simulink model "PFE_2Lignes_RNA (2)"  (R2024a)
settings: Solver=ode4  StartTime=0.0  StopTime=0.18  RelTol=1e-3
libraries: neural x202, spsRMSLib x12, spsThreePhasePISectionLineLib x4, spsThreePhaseFaultLib x2, spsThreePhaseVIMeasurementLib x2, spsThreePhaseSourceLib x2, spspowerguiLib x1
(part 3 of 10)

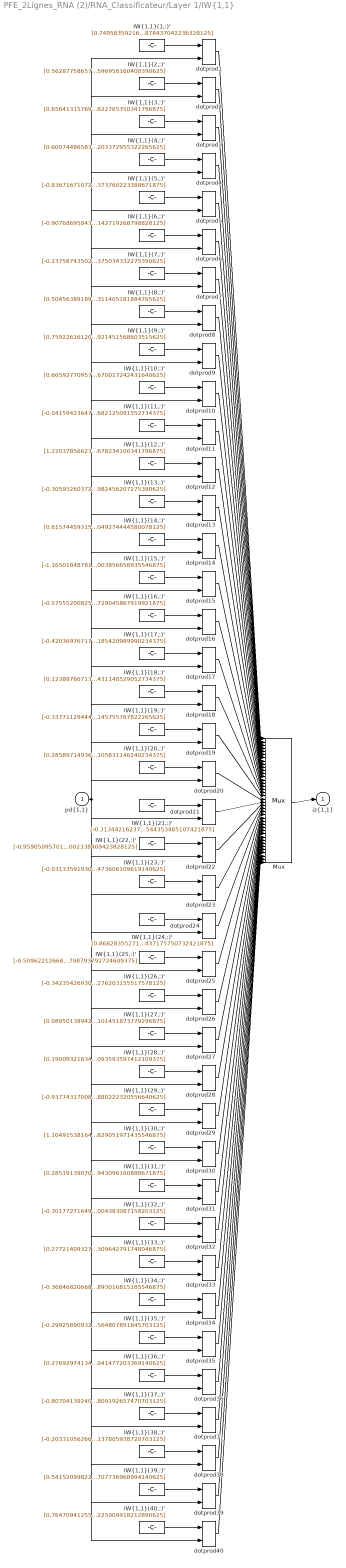
== system PFE_2Lignes_RNA (2)/RNA_Classificateur/Layer 1/IW{1,1} ==
  "pd{1,1}" : Inport  PortDimensions=12
      mask Display: e = 0.06;c1 = [120 230 180]/255;c2 = ([120 230 180]+0)/(256+128);c3 = ([120 230 180]+128)/(256+128);patch([0 1 1 0],[0 0 1 1],c1);patch([0 1 1 1-e 1-e 0+e],[0 0 1 1-e 0+e 0+e],c2);patch([0 0 1 1-e 0+e 0+e],[0 1 1 1-e 1-e 0+e],c3);plot([0 1 1 0 0],[0 0 1 1 0]);
  "IW{1,1}(1,:)'" : Constant  Value=[0.74958359216990821938253475309466011822223663330078125;-0.8029473672631188829740267465240322053432464599609375;-0.542336688026836544196385148097760975360870361328125;-0.787174648813282917814149186597205698490142822265625;0.5934798816135102850211069380748085677623748779296875;0.1866611157092597783613285855608410201966762542724609375;-0.408879266244710659616856673892471008002758026123046875;0.01913239052331479339574826781245064921677112579345703125;-0.106127660088452147046922391382395289838314056396484375;0.5668667292416820213674100159551016986370086669921875;-0.12326281029071710360067726242050412110984325408935546875;0.79123122581524285568121968026389367878437042236328125]
      mask Display: e = 0.06;c1 = [120 150 230]/255;c2 = ([120 150 230]+0)/383;c3 = ([120 150 230]+128)/383;patch([0 1 1 0],[0 0 1 1],c1);patch([0 1 1 1-e 1-e 0+e],[0 0 1 1-e 0+e 0+e],c2);patch([0 0 1 1-e 0+e 0+e],[0 1 1 1-e 1-e 0+e],c3);plot([0 1 1 0 0],[0 0 1 1 0]);disp('Weights');
  "IW{1,1}(10,:)'" : Constant  Value=[0.60592770957896824324251383586670272052288055419921875;-0.57064145847572245173751070979051291942596435546875;-0.57683424122696991265257793202181346714496612548828125;-1.4495291514928378973081635194830596446990966796875;-0.73466382714012545829262990082497708499431610107421875;-0.64755891681742239196495347641757689416408538818359375;-0.60153064759523289239950827322900295257568359375;-0.90205827349148481886231820681132376194000244140625;0.5948536687714207626953566432348452508449554443359375;-0.50297219156111128146591227050521411001682281494140625;1.567811975206783614567029871977865695953369140625;-0.252912599872824161995055192164727486670017242431640625]
      mask Display: e = 0.06;c1 = [120 150 230]/255;c2 = ([120 150 230]+0)/383;c3 = ([120 150 230]+128)/383;patch([0 1 1 0],[0 0 1 1],c1);patch([0 1 1 1-e 1-e 0+e],[0 0 1 1-e 0+e 0+e],c2);patch([0 0 1 1-e 0+e 0+e],[0 1 1 1-e 1-e 0+e],c3);plot([0 1 1 0 0],[0 0 1 1 0]);disp('Weights');
  "IW{1,1}(11,:)'" : Constant  Value=[-0.041594236471159569401567779323158902116119861602783203125;0.0541834052582221004090712312972755171358585357666015625;-1.2601601303957588040560722220106981694698333740234375;-2.32855835010428080522615346126258373260498046875;-1.3408389740320434402320870503899641335010528564453125;0.3734499673677518227776772619108669459819793701171875;0.5996288174482080624017044101492501795291900634765625;0.442299587174693920044177275485708378255367279052734375;-0.79910808052954729330252803265466354787349700927734375;-0.67576330904074810579373888685950078070163726806640625;1.6528925781939183270452531360206194221973419189453125;2.3480592220230303013295269920490682125091552734375]
      mask Display: e = 0.06;c1 = [120 150 230]/255;c2 = ([120 150 230]+0)/383;c3 = ([120 150 230]+128)/383;patch([0 1 1 0],[0 0 1 1],c1);patch([0 1 1 1-e 1-e 0+e],[0 0 1 1-e 0+e 0+e],c2);patch([0 0 1 1-e 0+e 0+e],[0 1 1 1-e 1-e 0+e],c3);plot([0 1 1 0 0],[0 0 1 1 0]);disp('Weights');
  "IW{1,1}(12,:)'" : Constant  Value=[1.2203785662394890376702960566035471856594085693359375;-0.08947721759545544661929028507074690423905849456787109375;-0.248432382462659473443267188486061058938503265380859375;-1.6836523036402055719662484989385120570659637451171875;1.8000899737378299736434428268694318830966949462890625;-0.324050010440849245441086168284527957439422607421875;1.327222054704254361467974376864731311798095703125;0.67379058195528285235553767051897011697292327880859375;-1.4433613727145309102439796333783306181430816650390625;-1.0976528220958334802759281956241466104984283447265625;0.2476851035413273616203611027231090702116489410400390625;1.6356974077387167465502670893329195678234100341796875]
      mask Display: e = 0.06;c1 = [120 150 230]/255;c2 = ([120 150 230]+0)/383;c3 = ([120 150 230]+128)/383;patch([0 1 1 0],[0 0 1 1],c1);patch([0 1 1 1-e 1-e 0+e],[0 0 1 1-e 0+e 0+e],c2);patch([0 0 1 1-e 0+e 0+e],[0 1 1 1-e 1-e 0+e],c3);plot([0 1 1 0 0],[0 0 1 1 0]);disp('Weights');
  "IW{1,1}(13,:)'" : Constant  Value=[-0.305952603724911120774976325265015475451946258544921875;0.2109724324184586163877241915542981587350368499755859375;-0.871724462567311508820466769975610077381134033203125;0.368499768652701009674643728430964983999729156494140625;0.246673658464245326715769124348298646509647369384765625;-0.442730444406182865879628707261872477829456329345703125;-1.096603408414358771238994449959136545658111572265625;0.434524950756032535270634298285585828125476837158203125;-0.3054258760453316678962210062309168279170989990234375;0.24218392291231183310884489401360042393207550048828125;0.8646470074893743973376558642485179007053375244140625;-0.1907281441165162017004064409775310195982456207275390625]
      mask Display: e = 0.06;c1 = [120 150 230]/255;c2 = ([120 150 230]+0)/383;c3 = ([120 150 230]+128)/383;patch([0 1 1 0],[0 0 1 1],c1);patch([0 1 1 1-e 1-e 0+e],[0 0 1 1-e 0+e 0+e],c2);patch([0 0 1 1-e 0+e 0+e],[0 1 1 1-e 1-e 0+e],c3);plot([0 1 1 0 0],[0 0 1 1 0]);disp('Weights');
  "IW{1,1}(14,:)'" : Constant  Value=[0.61574459315147722637817651047953404486179351806640625;-1.0623190979043048987051633957889862358570098876953125;0.394034092887489084677810069479164667427539825439453125;-2.248369712060643177409247073228470981121063232421875;0.5275119752705583753282780890003778040409088134765625;2.438367056160711143775188247673213481903076171875;0.22857017880371277573914312597480602562427520751953125;-1.0317290968902927961181603677687235176563262939453125;-0.2115671867019214003047267169677070342004299163818359375;-1.9027617943445609416386332668480463325977325439453125;0.60212334507071429978708465569070540368556976318359375;-0.82657639922626480188938558057998307049274444580078125]
      mask Display: e = 0.06;c1 = [120 150 230]/255;c2 = ([120 150 230]+0)/383;c3 = ([120 150 230]+128)/383;patch([0 1 1 0],[0 0 1 1],c1);patch([0 1 1 1-e 1-e 0+e],[0 0 1 1-e 0+e 0+e],c2);patch([0 0 1 1-e 0+e 0+e],[0 1 1 1-e 1-e 0+e],c3);plot([0 1 1 0 0],[0 0 1 1 0]);disp('Weights');
  "IW{1,1}(15,:)'" : Constant  Value=[-1.165018487811402270182270513032563030719757080078125;-0.1650855129048123537405245997433667071163654327392578125;-0.250310848664434038024495521312928758561611175537109375;0.367925209704279165823237462973338551819324493408203125;-1.053109213540988076118765093269757926464080810546875;1.1517107010752047902002459522918798029422760009765625;-0.5552091834027994554645601965603418648242950439453125;-0.56113154479276750041805144064710475504398345947265625;0.9146819847460303520847446634434163570404052734375;0.9900009386006491940435125798103399574756622314453125;-0.6463785661271843618891352889477275311946868896484375;-1.6172801313566320668968501195195131003856658935546875]
      mask Display: e = 0.06;c1 = [120 150 230]/255;c2 = ([120 150 230]+0)/383;c3 = ([120 150 230]+128)/383;patch([0 1 1 0],[0 0 1 1],c1);patch([0 1 1 1-e 1-e 0+e],[0 0 1 1-e 0+e 0+e],c2);patch([0 0 1 1-e 0+e 0+e],[0 1 1 1-e 1-e 0+e],c3);plot([0 1 1 0 0],[0 0 1 1 0]);disp('Weights');
  "IW{1,1}(16,:)'" : Constant  Value=[-0.57555200825379848605933830185676924884319305419921875;0.1994373147096829279600882500744774006307125091552734375;-0.412238082672211680890228535645292140543460845947265625;-0.42438555031721836297009531335788778960704803466796875;-0.93932452660136644961852425694814883172512054443359375;0.51360222841409786109778679019655101001262664794921875;0.1309899446070415252041385656411875970661640167236328125;-0.182257806815278977641270330423139967024326324462890625;0.8509013471342818935028162741218693554401397705078125;-0.388818754819776180031709600370959378778934478759765625;-1.025285492360808348166756331920623779296875;-0.203483170274558755608040883089415729045867919921875]
      mask Display: e = 0.06;c1 = [120 150 230]/255;c2 = ([120 150 230]+0)/383;c3 = ([120 150 230]+128)/383;patch([0 1 1 0],[0 0 1 1],c1);patch([0 1 1 1-e 1-e 0+e],[0 0 1 1-e 0+e 0+e],c2);patch([0 0 1 1-e 0+e 0+e],[0 1 1 1-e 1-e 0+e],c3);plot([0 1 1 0 0],[0 0 1 1 0]);disp('Weights');
  "IW{1,1}(17,:)'" : Constant  Value=[-0.420369767179770204013067314008367247879505157470703125;-0.64126174661276513777607988231466151773929595947265625;-0.388206694327405232858296812992193736135959625244140625;0.79635997694663307466811374979442916810512542724609375;0.60879685212660639148651853247429244220256805419921875;-0.591923664374563340828672153293155133724212646484375;0.1847453299443102270327443648056942038238048553466796875;-0.292667915200633343975056277486146427690982818603515625;-0.93611854779757319722222064228844828903675079345703125;0.2289312304159379085621850435927626676857471466064453125;0.477672003545131840240856035961769521236419677734375;-0.5429342609145473286247352007194422185420989990234375]
      mask Display: e = 0.06;c1 = [120 150 230]/255;c2 = ([120 150 230]+0)/383;c3 = ([120 150 230]+128)/383;patch([0 1 1 0],[0 0 1 1],c1);patch([0 1 1 1-e 1-e 0+e],[0 0 1 1-e 0+e 0+e],c2);patch([0 0 1 1-e 0+e 0+e],[0 1 1 1-e 1-e 0+e],c3);plot([0 1 1 0 0],[0 0 1 1 0]);disp('Weights');
  "IW{1,1}(18,:)'" : Constant  Value=[0.1238876071364114761497177141791325993835926055908203125;-0.77572554113254332808224944528774358332157135009765625;-0.08898063744331276281318565679612220264971256256103515625;1.57613590534866698789073780062608420848846435546875;0.2321005336110762706791632581371231935918331146240234375;-0.73676696655795925749998787068761885166168212890625;0.142658166835522681736847516731359064579010009765625;0.5747450524492887513616778960567899048328399658203125;-1.105370078416131551790613229968585073947906494140625;-2.21704492450396539737766943289898335933685302734375;1.0876593267347447469006738174357451498508453369140625;-0.72611976053770399541775759644224308431148529052734375]
      mask Display: e = 0.06;c1 = [120 150 230]/255;c2 = ([120 150 230]+0)/383;c3 = ([120 150 230]+128)/383;patch([0 1 1 0],[0 0 1 1],c1);patch([0 1 1 1-e 1-e 0+e],[0 0 1 1-e 0+e 0+e],c2);patch([0 0 1 1-e 0+e 0+e],[0 1 1 1-e 1-e 0+e],c3);plot([0 1 1 0 0],[0 0 1 1 0]);disp('Weights');
  "IW{1,1}(19,:)'" : Constant  Value=[-0.33771129444509118133765923630562610924243927001953125;0.0713367915505468130898947265450260601937770843505859375;0.2057896003228630033010659872161340899765491485595703125;2.20019744077431322892834941740147769451141357421875;-2.278663430987770244229295713012106716632843017578125;1.0768853464076302284269104347913525998592376708984375;-0.90948100032295198236198530139517970383167266845703125;1.2699892475521668000482122806715779006481170654296875;-0.374919053331535356843318140818155370652675628662109375;0.63267481864128505275601810353691689670085906982421875;-2.264524629934004718023743407684378325939178466796875;0.325611439903700505826833477840409614145755767822265625]
      mask Display: e = 0.06;c1 = [120 150 230]/255;c2 = ([120 150 230]+0)/383;c3 = ([120 150 230]+128)/383;patch([0 1 1 0],[0 0 1 1],c1);patch([0 1 1 1-e 1-e 0+e],[0 0 1 1-e 0+e 0+e],c2);patch([0 0 1 1-e 0+e 0+e],[0 1 1 1-e 1-e 0+e],c3);plot([0 1 1 0 0],[0 0 1 1 0]);disp('Weights');
  "IW{1,1}(2,:)'" : Constant  Value=[0.56287758657184328026090724961250089108943939208984375;0.62349868963765164853185751780983991920948028564453125;0.439815094086207059032034294432378374040126800537109375;0.47907287682830890229723763695801608264446258544921875;-0.209879774707502075870024782489053905010223388671875;-0.14745846190329292557663620755192823708057403564453125;-0.882701370669022100656775364768691360950469970703125;-0.7129252832091104163936279292101971805095672607421875;-0.76504800874029665891384865972213447093963623046875;-0.674348859168129255436952007585205137729644775390625;0.12273009441098824134908085170536651276051998138427734375;0.0229431755667083604743883284982075565494596958160400390625]
      mask Display: e = 0.06;c1 = [120 150 230]/255;c2 = ([120 150 230]+0)/383;c3 = ([120 150 230]+128)/383;patch([0 1 1 0],[0 0 1 1],c1);patch([0 1 1 1-e 1-e 0+e],[0 0 1 1-e 0+e 0+e],c2);patch([0 0 1 1-e 0+e 0+e],[0 1 1 1-e 1-e 0+e],c3);plot([0 1 1 0 0],[0 0 1 1 0]);disp('Weights');
  "IW{1,1}(20,:)'" : Constant  Value=[0.285897149366284797356030367154744453728199005126953125;-1.071211066211320339647272703587077558040618896484375;1.042160099435808451318052902934141457080841064453125;0.7370117529808191125795246989582665264606475830078125;-1.5106532728405495102919076089165173470973968505859375;-2.101314330452319634190416763885878026485443115234375;-0.0824484752168814782891104187001474201679229736328125;-1.1490974138089724565503502162755466997623443603515625;0.429340350947707449780210708922822959721088409423828125;1.6983804194670313325588040243019349873065948486328125;-0.6343565826158401588230617562658153474330902099609375;0.77783500854026621507131267208023928105831146240234375]
      mask Display: e = 0.06;c1 = [120 150 230]/255;c2 = ([120 150 230]+0)/383;c3 = ([120 150 230]+128)/383;patch([0 1 1 0],[0 0 1 1],c1);patch([0 1 1 1-e 1-e 0+e],[0 0 1 1-e 0+e 0+e],c2);patch([0 0 1 1-e 0+e 0+e],[0 1 1 1-e 1-e 0+e],c3);plot([0 1 1 0 0],[0 0 1 1 0]);disp('Weights');
  "IW{1,1}(21,:)'" : Constant  Value=[-0.313442162370461574472102483923663385212421417236328125;0.71069365723408439716735074398457072675228118896484375;0.7368025277872487510677501632017083466053009033203125;0.250940337360686938072973362068296410143375396728515625;0.36219419785523376820179919377551414072513580322265625;-0.045125177484137184158452527071858639828860759735107421875;-0.9373772040546857198251018417067825794219970703125;-0.8005469342332072191226188806467689573764801025390625;0.479706543742673463537329325845348648726940155029296875;-0.489203575067028051392981069511733949184417724609375;0.89499756815461750658613482301007024943828582763671875;-0.9393115987438498404316078449483029544353485107421875]
      mask Display: e = 0.06;c1 = [120 150 230]/255;c2 = ([120 150 230]+0)/383;c3 = ([120 150 230]+128)/383;patch([0 1 1 0],[0 0 1 1],c1);patch([0 1 1 1-e 1-e 0+e],[0 0 1 1-e 0+e 0+e],c2);patch([0 0 1 1-e 0+e 0+e],[0 1 1 1-e 1-e 0+e],c3);plot([0 1 1 0 0],[0 0 1 1 0]);disp('Weights');
  "IW{1,1}(22,:)'" : Constant  Value=[-0.9590509570193808119853429161594249308109283447265625;-0.493730940753906055729061108650057576596736907958984375;-0.8050191480991275572165477569797076284885406494140625;-0.28324115064341359726540758856572210788726806640625;-0.0855579308944639238543317105722962878644466400146484375;-0.2982589814017286844460841166437603533267974853515625;0.8651890058906144265193915998679585754871368408203125;-0.2127697372929893138149282094673253595829010009765625;-0.2118629696150977348434452096626046113669872283935546875;0.614617181476534657491583857336081564426422119140625;0.5175871796669948565750019042752683162689208984375;0.283420043030612689438640927619417198002338409423828125]
      mask Display: e = 0.06;c1 = [120 150 230]/255;c2 = ([120 150 230]+0)/383;c3 = ([120 150 230]+128)/383;patch([0 1 1 0],[0 0 1 1],c1);patch([0 1 1 1-e 1-e 0+e],[0 0 1 1-e 0+e 0+e],c2);patch([0 0 1 1-e 0+e 0+e],[0 1 1 1-e 1-e 0+e],c3);plot([0 1 1 0 0],[0 0 1 1 0]);disp('Weights');
  "IW{1,1}(23,:)'" : Constant  Value=[-0.031335919302591545843039710916855256073176860809326171875;-0.264118888374587523770742336637340486049652099609375;-0.99437742834595932439611942754709161818027496337890625;-0.48613182289601153396318977684131823480129241943359375;-0.65349579829228721106204602619982324540615081787109375;-0.82571376926229722581496162092662416398525238037109375;0.2174726698576462113887686200541793368756771087646484375;-0.73776313034045315486508798130671493709087371826171875;0.7378956287314346607075776773854158818721771240234375;-0.021332740476675084162483386762687587179243564605712890625;0.22149884534648800471501317588263191282749176025390625;0.86225703326549807403722525123157538473606109619140625]
      mask Display: e = 0.06;c1 = [120 150 230]/255;c2 = ([120 150 230]+0)/383;c3 = ([120 150 230]+128)/383;patch([0 1 1 0],[0 0 1 1],c1);patch([0 1 1 1-e 1-e 0+e],[0 0 1 1-e 0+e 0+e],c2);patch([0 0 1 1-e 0+e 0+e],[0 1 1 1-e 1-e 0+e],c3);plot([0 1 1 0 0],[0 0 1 1 0]);disp('Weights');
  "IW{1,1}(24,:)'" : Constant  Value=[0.8682835527171566258886059586075134575366973876953125;-0.338032804470147107966937483070068992674350738525390625;0.42663950553967155965295887654065154492855072021484375;0.07994886852322703740814091588617884553968906402587890625;-0.08234018636647570665854090066204662434756755828857421875;-0.56246234595990518556618553702719509601593017578125;-0.87800269121447815923175994612392969429492950439453125;0.67292433346952262862572524682036601006984710693359375;0.35843044089265407858846401722985319793224334716796875;-0.01037903761493451197661652685155786457471549510955810546875;0.419685343853191117347023464390076696872711181640625;0.82952182259364171112991925838286988437175750732421875]
      mask Display: e = 0.06;c1 = [120 150 230]/255;c2 = ([120 150 230]+0)/383;c3 = ([120 150 230]+128)/383;patch([0 1 1 0],[0 0 1 1],c1);patch([0 1 1 1-e 1-e 0+e],[0 0 1 1-e 0+e 0+e],c2);patch([0 0 1 1-e 0+e 0+e],[0 1 1 1-e 1-e 0+e],c3);plot([0 1 1 0 0],[0 0 1 1 0]);disp('Weights');
  "IW{1,1}(25,:)'" : Constant  Value=[-0.5096221266848035558183482862659730017185211181640625;-0.33408111078061530907490350728039629757404327392578125;0.053466115900446635478271417696305434219539165496826171875;-0.4334640772843945111247876411653123795986175537109375;-1.11725240942251868858647867455147206783294677734375;-0.8929572284339248877671479931450448930263519287109375;-0.2012255857319280305528508279166999273002147674560546875;-0.5698313421375633680554528837092220783233642578125;-0.7647545897762022537591519721900112926959991455078125;-0.25538460783435545931041588119114749133586883544921875;-0.353646046014701231907650935681886039674282073974609375;0.354005086921495182306074411826557479798793792724609375]
      mask Display: e = 0.06;c1 = [120 150 230]/255;c2 = ([120 150 230]+0)/383;c3 = ([120 150 230]+128)/383;patch([0 1 1 0],[0 0 1 1],c1);patch([0 1 1 1-e 1-e 0+e],[0 0 1 1-e 0+e 0+e],c2);patch([0 0 1 1-e 0+e 0+e],[0 1 1 1-e 1-e 0+e],c3);plot([0 1 1 0 0],[0 0 1 1 0]);disp('Weights');
  "IW{1,1}(26,:)'" : Constant  Value=[-0.3423542693008467807658234960399568080902099609375;-0.65877052593968421501102739057387225329875946044921875;0.393800774596241687230957495557959191501140594482421875;-1.1600315330827519755274579438264481723308563232421875;-0.71438883033852540460628688379074446856975555419921875;0.161594455696278116452191397911519743502140045166015625;-0.595002607394423232989311145502142608165740966796875;0.53582780307071098402360576073988340795040130615234375;-0.2830443249472971434244072952424176037311553955078125;0.2438679104402185771061084551547537557780742645263671875;0.8530165391517396944465190244955010712146759033203125;-0.477263046162692383678205487740342505276203155517578125]
      mask Display: e = 0.06;c1 = [120 150 230]/255;c2 = ([120 150 230]+0)/383;c3 = ([120 150 230]+128)/383;patch([0 1 1 0],[0 0 1 1],c1);patch([0 1 1 1-e 1-e 0+e],[0 0 1 1-e 0+e 0+e],c2);patch([0 0 1 1-e 0+e 0+e],[0 1 1 1-e 1-e 0+e],c3);plot([0 1 1 0 0],[0 0 1 1 0]);disp('Weights');
  "IW{1,1}(27,:)'" : Constant  Value=[0.08950138942217437942883151436035404913127422332763671875;1.3685401924282574182001326335011981427669525146484375;-0.288351551229408753496130657367757521569728851318359375;-0.71976588579313471871756746622850187122821807861328125;-0.52243867576969871269199074959033168852329254150390625;2.612100797819043140890471477177925407886505126953125;-1.27054609389886774550859627197496592998504638671875;1.4995893391046692944001961222966201603412628173828125;-0.099707396420515903567860505063435994088649749755859375;1.2431004909587823892280766813200898468494415283203125;-0.64312205526082066864290709418128244578838348388671875;-0.10866294126831392563570233278369414620101451873779296875]
      mask Display: e = 0.06;c1 = [120 150 230]/255;c2 = ([120 150 230]+0)/383;c3 = ([120 150 230]+128)/383;patch([0 1 1 0],[0 0 1 1],c1);patch([0 1 1 1-e 1-e 0+e],[0 0 1 1-e 0+e 0+e],c2);patch([0 0 1 1-e 0+e 0+e],[0 1 1 1-e 1-e 0+e],c3);plot([0 1 1 0 0],[0 0 1 1 0]);disp('Weights');
  "IW{1,1}(28,:)'" : Constant  Value=[0.190093216345575910519727358405361883342266082763671875;0.3459347222775852603859902956173755228519439697265625;0.1488544304146839636349142210747231729328632354736328125;-0.84436799503464687877141159333405084908008575439453125;-0.043616504441921312429375490182792418636381626129150390625;-0.406650868392631481551546812625019811093807220458984375;-0.6335629077808870857069223347934894263744354248046875;-0.1333311244937185613412822249301825650036334991455078125;-0.38599030556140478953608408119180239737033843994140625;-0.03760225945764107680080456930227228440344333648681640625;1.0547147290717828749251339104375801980495452880859375;-0.8816665448833267415551517842686735093593597412109375]
      mask Display: e = 0.06;c1 = [120 150 230]/255;c2 = ([120 150 230]+0)/383;c3 = ([120 150 230]+128)/383;patch([0 1 1 0],[0 0 1 1],c1);patch([0 1 1 1-e 1-e 0+e],[0 0 1 1-e 0+e 0+e],c2);patch([0 0 1 1-e 0+e 0+e],[0 1 1 1-e 1-e 0+e],c3);plot([0 1 1 0 0],[0 0 1 1 0]);disp('Weights');
  "IW{1,1}(29,:)'" : Constant  Value=[-0.9377431700885920928811856356333009898662567138671875;-0.41871014072329704180930320944753475487232208251953125;-0.30656734193459700410500090583809651434421539306640625;0.48579727512091064323129785407218150794506072998046875;0.568634796685665744320203884853981435298919677734375;0.041760693543964326479578375028722803108394145965576171875;0.50950195077496907014591442930395714938640594482421875;0.62995217911531053989193651432287879288196563720703125;0.465545832022614458622911115526221692562103271484375;0.93160272044449976558411208316101692616939544677734375;0.455869667774234266222066480622743256390094757080078125;0.07025705649596970803205664424240239895880222320556640625]
      mask Display: e = 0.06;c1 = [120 150 230]/255;c2 = ([120 150 230]+0)/383;c3 = ([120 150 230]+128)/383;patch([0 1 1 0],[0 0 1 1],c1);patch([0 1 1 1-e 1-e 0+e],[0 0 1 1-e 0+e 0+e],c2);patch([0 0 1 1-e 0+e 0+e],[0 1 1 1-e 1-e 0+e],c3);plot([0 1 1 0 0],[0 0 1 1 0]);disp('Weights');
  "IW{1,1}(3,:)'" : Constant  Value=[0.65641315769168706584224537436966784298419952392578125;0.95965783508391699907491556587046943604946136474609375;-0.2152247721630420607130673715801094658672809600830078125;0.317281125122891249912271405264618806540966033935546875;-0.61078832199027666138846370813553221523761749267578125;0.10949722031622351192670095088033122010529041290283203125;0.1124212875620385909680720715186907909810543060302734375;0.74937070531208183066240735570318065583705902099609375;0.7614081896496200929647102384478785097599029541015625;-0.416611934081368151527868803896126337349414825439453125;0.7932555092323492207384560970240272581577301025390625;0.89911069595746351268417129176668822765350341796875]
      mask Display: e = 0.06;c1 = [120 150 230]/255;c2 = ([120 150 230]+0)/383;c3 = ([120 150 230]+128)/383;patch([0 1 1 0],[0 0 1 1],c1);patch([0 1 1 1-e 1-e 0+e],[0 0 1 1-e 0+e 0+e],c2);patch([0 0 1 1-e 0+e 0+e],[0 1 1 1-e 1-e 0+e],c3);plot([0 1 1 0 0],[0 0 1 1 0]);disp('Weights');
  "IW{1,1}(30,:)'" : Constant  Value=[1.1049153816467895961039857866126112639904022216796875;-0.53997558976443393863320352465962059795856475830078125;-0.29341557443190480203298875494510866701602935791015625;-1.281561303027391129916168210911564528942108154296875;-1.5163694776935543462315081342239864170551300048828125;2.712509809409909156130424889852292835712432861328125;0.492131681291292644164769853887264616787433624267578125;0.174527918481056143473750807970645837485790252685546875;-0.349498727995869173934551099591772072017192840576171875;0.59797003361281808597738063326687552034854888916015625;0.83240948658350488731372252004803158342838287353515625;-0.05640705661161364570244103333607199601829051971435546875]
      mask Display: e = 0.06;c1 = [120 150 230]/255;c2 = ([120 150 230]+0)/383;c3 = ([120 150 230]+128)/383;patch([0 1 1 0],[0 0 1 1],c1);patch([0 1 1 1-e 1-e 0+e],[0 0 1 1-e 0+e 0+e],c2);patch([0 0 1 1-e 0+e 0+e],[0 1 1 1-e 1-e 0+e],c3);plot([0 1 1 0 0],[0 0 1 1 0]);disp('Weights');
  "IW{1,1}(31,:)'" : Constant  Value=[0.28519139070568699789731681448756717145442962646484375;-1.862443606980191734834306771517731249332427978515625;0.8013557171435683468274646656936965882778167724609375;1.1042674905459006762242779586813412606716156005859375;0.16541559268416694550296597299166023731231689453125;0.1831329137039820753596330860091256909072399139404296875;0.451396702089381818279179015007684938609600067138671875;-0.222687383867321175845432890127995051443576812744140625;1.629423175853772054466617191792465746402740478515625;-0.57012463147081238190594376646913588047027587890625;2.21204921457433467679720706655643880367279052734375;-2.8511850436189671853526306222192943096160888671875]
      mask Display: e = 0.06;c1 = [120 150 230]/255;c2 = ([120 150 230]+0)/383;c3 = ([120 150 230]+128)/383;patch([0 1 1 0],[0 0 1 1],c1);patch([0 1 1 1-e 1-e 0+e],[0 0 1 1-e 0+e 0+e],c2);patch([0 0 1 1-e 0+e 0+e],[0 1 1 1-e 1-e 0+e],c3);plot([0 1 1 0 0],[0 0 1 1 0]);disp('Weights');
  "IW{1,1}(32,:)'" : Constant  Value=[-0.301772716498337700841148034669458866119384765625;-0.414429934390460219528762308982550166547298431396484375;0.1380777058785409849850367436374654062092304229736328125;-0.7143244134519781685099815149442292749881744384765625;-0.77940794840309080004914221717626787722110748291015625;-1.2428186126836837654963119348394684493541717529296875;-0.391212337652795338893696452942094765603542327880859375;0.475034841084361392216095509866136126220226287841796875;-0.4299337892150332240959187402040697634220123291015625;-0.6281549902762579851156488075503148138523101806640625;1.060508076003738864301340072415769100189208984375;0.485821416719840915021677574259229004383087158203125]
      mask Display: e = 0.06;c1 = [120 150 230]/255;c2 = ([120 150 230]+0)/383;c3 = ([120 150 230]+128)/383;patch([0 1 1 0],[0 0 1 1],c1);patch([0 1 1 1-e 1-e 0+e],[0 0 1 1-e 0+e 0+e],c2);patch([0 0 1 1-e 0+e 0+e],[0 1 1 1-e 1-e 0+e],c3);plot([0 1 1 0 0],[0 0 1 1 0]);disp('Weights');
  "IW{1,1}(33,:)'" : Constant  Value=[0.277214093272214301411082715276279486715793609619140625;-0.92575351685280027336233388268738053739070892333984375;-0.94168797078716626192118610561010427772998809814453125;0.434861051287833533240956285226275213062763214111328125;-0.580249336840946927651430087280459702014923095703125;-0.379448799341846887411833222358836792409420013427734375;-0.008056916678392180009016243502628640271723270416259765625;0.838796765298734481319797851028852164745330810546875;-0.1206418706210981850457386599373421631753444671630859375;-0.1670855221535699486334891616934328339993953704833984375;-0.476500419080890302847564043986494652926921844482421875;0.529235878067051412898536000284366309642791748046875]
      mask Display: e = 0.06;c1 = [120 150 230]/255;c2 = ([120 150 230]+0)/383;c3 = ([120 150 230]+128)/383;patch([0 1 1 0],[0 0 1 1],c1);patch([0 1 1 1-e 1-e 0+e],[0 0 1 1-e 0+e 0+e],c2);patch([0 0 1 1-e 0+e 0+e],[0 1 1 1-e 1-e 0+e],c3);plot([0 1 1 0 0],[0 0 1 1 0]);disp('Weights');
  "IW{1,1}(34,:)'" : Constant  Value=[-0.3684682066801336919326104180072434246540069580078125;-0.6352643746280903780387916413019411265850067138671875;0.70922280885724386934043650398962199687957763671875;0.57918446406515367019807172255241312086582183837890625;-0.0775289597604681690601324817180284298956394195556640625;0.7739422565547275922881453880108892917633056640625;0.69494552120529384797720240385388024151325225830078125;-0.319218125764637761232478396777878515422344207763671875;0.57296390287849618960791531208087690174579620361328125;-0.0858820073557324814572666582535021007061004638671875;-0.056006971209040086467911834233746048994362354278564453125;0.859022811903467964356195807340554893016815185546875]
      mask Display: e = 0.06;c1 = [120 150 230]/255;c2 = ([120 150 230]+0)/383;c3 = ([120 150 230]+128)/383;patch([0 1 1 0],[0 0 1 1],c1);patch([0 1 1 1-e 1-e 0+e],[0 0 1 1-e 0+e 0+e],c2);patch([0 0 1 1-e 0+e 0+e],[0 1 1 1-e 1-e 0+e],c3);plot([0 1 1 0 0],[0 0 1 1 0]);disp('Weights');
  "IW{1,1}(35,:)'" : Constant  Value=[-0.299258909321519162016755899458075873553752899169921875;0.2966388415741152417837156463065184652805328369140625;1.018171120787297656562486736220307648181915283203125;-1.124625556509126766968620358966290950775146484375;-1.439779048212390666350302126375027000904083251953125;0.86076943642049152938255929257138632237911224365234375;-0.83449722454053343323465696812490932643413543701171875;0.85754039690351591129768848986714147031307220458984375;-0.50045011901598346337749489975976757705211639404296875;0.243723327944616041662584393634460866451263427734375;1.16440210158013979224733702722005546092987060546875;-0.586932156418353390137099268031306564807891845703125]
      mask Display: e = 0.06;c1 = [120 150 230]/255;c2 = ([120 150 230]+0)/383;c3 = ([120 150 230]+128)/383;patch([0 1 1 0],[0 0 1 1],c1);patch([0 1 1 1-e 1-e 0+e],[0 0 1 1-e 0+e 0+e],c2);patch([0 0 1 1-e 0+e 0+e],[0 1 1 1-e 1-e 0+e],c3);plot([0 1 1 0 0],[0 0 1 1 0]);disp('Weights');
  "IW{1,1}(36,:)'" : Constant  Value=[0.27692974134838854727291845847503282129764556884765625;0.77329622179783275015552135300822556018829345703125;-0.1675059555554003765109882806427776813507080078125;-0.89453860910611260326419369448558427393436431884765625;0.135909151123754623480266445767483673989772796630859375;-0.395709438384614475836542624165304005146026611328125;0.429729256934494541209090812117210589349269866943359375;0.74666018683282786572164013705332763493061065673828125;-0.3527021687177949171854152154992334544658660888671875;0.3362811681978075117882553968229331076145172119140625;-0.89909554477031738972669927534298039972782135009765625;-0.21445098130394557589539772379794158041477203369140625]
      mask Display: e = 0.06;c1 = [120 150 230]/255;c2 = ([120 150 230]+0)/383;c3 = ([120 150 230]+128)/383;patch([0 1 1 0],[0 0 1 1],c1);patch([0 1 1 1-e 1-e 0+e],[0 0 1 1-e 0+e 0+e],c2);patch([0 0 1 1-e 0+e 0+e],[0 1 1 1-e 1-e 0+e],c3);plot([0 1 1 0 0],[0 0 1 1 0]);disp('Weights');
  "IW{1,1}(37,:)'" : Constant  Value=[-0.80704139240025274393275367401656694710254669189453125;-0.25956215745037225506308686817646957933902740478515625;0.062075476078189729955969511365765356458723545074462890625;-0.325749693859563371756138394630397669970989227294921875;0.048574291467453123427588934646337293088436126708984375;0.89002497988019191321740208877599798142910003662109375;0.65323639460772664477872240240685641765594482421875;0.473597836610536393475712202416616491973400115966796875;-0.6069538552713442669528376427479088306427001953125;0.71567198082631888755855698036612011492252349853515625;-0.57652578697549572428471265084226615726947784423828125;0.0968309675838574801520763912776601500809192657470703125]
      mask Display: e = 0.06;c1 = [120 150 230]/255;c2 = ([120 150 230]+0)/383;c3 = ([120 150 230]+128)/383;patch([0 1 1 0],[0 0 1 1],c1);patch([0 1 1 1-e 1-e 0+e],[0 0 1 1-e 0+e 0+e],c2);patch([0 0 1 1-e 0+e 0+e],[0 1 1 1-e 1-e 0+e],c3);plot([0 1 1 0 0],[0 0 1 1 0]);disp('Weights');
  "IW{1,1}(38,:)'" : Constant  Value=[-0.203310562661204674572701378565398044884204864501953125;0.1788840987199529497519989718057331629097461700439453125;0.59513101026308756757998708053492009639739990234375;0.62350590814322259802793269045650959014892578125;1.8690381951598677989778707342338748276233673095703125;0.033032499657993895370022841007084934972226619720458984375;0.1757252254517237821662689611912355758249759674072265625;0.376049872023515752150757407434866763651371002197265625;0.69247672917727165486923013304476626217365264892578125;-1.2965395534711678937611623041448183357715606689453125;-0.93997399702286477118917673578835092484951019287109375;-0.6158625098382881635217245275271125137805938720703125]
      mask Display: e = 0.06;c1 = [120 150 230]/255;c2 = ([120 150 230]+0)/383;c3 = ([120 150 230]+128)/383;patch([0 1 1 0],[0 0 1 1],c1);patch([0 1 1 1-e 1-e 0+e],[0 0 1 1-e 0+e 0+e],c2);patch([0 0 1 1-e 0+e 0+e],[0 1 1 1-e 1-e 0+e],c3);plot([0 1 1 0 0],[0 0 1 1 0]);disp('Weights');
  "IW{1,1}(39,:)'" : Constant  Value=[0.54152099822578259047389792613103054463863372802734375;0.160174799891083907699140809199889190495014190673828125;-0.265786400862816851731196265973267145454883575439453125;-0.438811475002850170934465268146595917642116546630859375;0.39802426181648675740376575049594976007938385009765625;-0.686630434166221714775701912003569304943084716796875;-0.6962055175771599824230406738934107124805450439453125;1.040406774592970595705310188350267708301544189453125;-0.1016401613938503756262576871449709869921207427978515625;-0.10287828002409356298318954259229940362274646759033203125;-0.89655346696509052861756572383455932140350341796875;0.1339360030076012508803984246696927584707736968994140625]
      mask Display: e = 0.06;c1 = [120 150 230]/255;c2 = ([120 150 230]+0)/383;c3 = ([120 150 230]+128)/383;patch([0 1 1 0],[0 0 1 1],c1);patch([0 1 1 1-e 1-e 0+e],[0 0 1 1-e 0+e 0+e],c2);patch([0 0 1 1-e 0+e 0+e],[0 1 1 1-e 1-e 0+e],c3);plot([0 1 1 0 0],[0 0 1 1 0]);disp('Weights');
  "IW{1,1}(4,:)'" : Constant  Value=[0.600744865837338437586367945186793804168701171875;0.81736400318501434281159845340880565345287322998046875;0.96733501205360805652588851444306783378124237060546875;-0.60862859040623795703339737883652560412883758544921875;-0.89272101877643417200403064271085895597934722900390625;0.1445345695507280481262313287516008131206035614013671875;0.740054999198556995310127604170702397823333740234375;0.040437384319956602707346604574922821484506130218505859375;-0.1211526191911180549976023712588357739150524139404296875;-0.15047732920444889526123688483494333922863006591796875;-0.374151436983826968241118038349668495357036590576171875;-0.83178145689704996446067752913222648203372955322265625]
      mask Display: e = 0.06;c1 = [120 150 230]/255;c2 = ([120 150 230]+0)/383;c3 = ([120 150 230]+128)/383;patch([0 1 1 0],[0 0 1 1],c1);patch([0 1 1 1-e 1-e 0+e],[0 0 1 1-e 0+e 0+e],c2);patch([0 0 1 1-e 0+e 0+e],[0 1 1 1-e 1-e 0+e],c3);plot([0 1 1 0 0],[0 0 1 1 0]);disp('Weights');
  "IW{1,1}(40,:)'" : Constant  Value=[0.76470941255774160794089766568504273891448974609375;0.7509352048436939153219782383530400693416595458984375;0.66737230266155267432992559406557120382785797119140625;0.48756201808471200109806886757723987102508544921875;-0.58779814708604904982536254465230740606784820556640625;-0.290634263261388692267672695379587821662425994873046875;-0.52771118724632148921926955154049210250377655029296875;-0.3148389528275117310585073937545530498027801513671875;0.57937948246702497545612686735694296658039093017578125;-0.171738803664202688281648079282604157924652099609375;0.3012940300772226631664807428023777902126312255859375;0.55218816944886450759355511763715185225009918212890625]
      mask Display: e = 0.06;c1 = [120 150 230]/255;c2 = ([120 150 230]+0)/383;c3 = ([120 150 230]+128)/383;patch([0 1 1 0],[0 0 1 1],c1);patch([0 1 1 1-e 1-e 0+e],[0 0 1 1-e 0+e 0+e],c2);patch([0 0 1 1-e 0+e 0+e],[0 1 1 1-e 1-e 0+e],c3);plot([0 1 1 0 0],[0 0 1 1 0]);disp('Weights');
  "IW{1,1}(5,:)'" : Constant  Value=[-0.836716710720950995749944922863505780696868896484375;0.439411125451092399174513047910295426845550537109375;-0.1971139720063680711437115178341628052294254302978515625;-1.1003131078183823188254564229282550513744354248046875;0.02851888725345029518276618318850523792207241058349609375;-2.07109382987704382372839972958900034427642822265625;0.041456430285719471362515520240776822902262210845947265625;-0.65475871116475203859152998120407573878765106201171875;0.73798542834985292326877015511854551732540130615234375;1.375145340437987417914200705126859247684478759765625;1.914784300795295823860442396835424005985260009765625;0.95842545149267521775726663690875284373760223388671875]
      mask Display: e = 0.06;c1 = [120 150 230]/255;c2 = ([120 150 230]+0)/383;c3 = ([120 150 230]+128)/383;patch([0 1 1 0],[0 0 1 1],c1);patch([0 1 1 1-e 1-e 0+e],[0 0 1 1-e 0+e 0+e],c2);patch([0 0 1 1-e 0+e 0+e],[0 1 1 1-e 1-e 0+e],c3);plot([0 1 1 0 0],[0 0 1 1 0]);disp('Weights');
  "IW{1,1}(6,:)'" : Constant  Value=[-0.90768695843270974510375026511610485613346099853515625;-0.68351866834691554775105259977863170206546783447265625;1.2551835000960258614810527433292008936405181884765625;0.70545498306578269254174529123702086508274078369140625;-2.12807959265498336520749944611452519893646240234375;0.497168630609090722582976695775869302451610565185546875;-0.208328719791111061088173528332845307886600494384765625;0.1446092901230397742562416851797024719417095184326171875;-0.20704854405500150438257378482376225292682647705078125;2.448444622861401409608106405357830226421356201171875;-0.84050738810234004727561796244117431342601776123046875;0.039472385311477516112166341599731822498142719268798828125]
      mask Display: e = 0.06;c1 = [120 150 230]/255;c2 = ([120 150 230]+0)/383;c3 = ([120 150 230]+128)/383;patch([0 1 1 0],[0 0 1 1],c1);patch([0 1 1 1-e 1-e 0+e],[0 0 1 1-e 0+e 0+e],c2);patch([0 0 1 1-e 0+e 0+e],[0 1 1 1-e 1-e 0+e],c3);plot([0 1 1 0 0],[0 0 1 1 0]);disp('Weights');
  "IW{1,1}(7,:)'" : Constant  Value=[-0.237587435025801596566452644765377044677734375;0.94238608006865531852014328251243568956851959228515625;0.7885322751371912630702354363165795803070068359375;-0.1640548008439850768969137106978450901806354522705078125;-0.89611334097657946440307341617881320416927337646484375;0.0029081416154285743592977642180130715132690966129302978515625;-0.49500699678215998034147560247220098972320556640625;-0.457738654151404744663267365467618219554424285888671875;-0.354984270142353341981333869625814259052276611328125;-0.477987001565870428532178948444197885692119598388671875;0.00767064224277644833571709881425704224966466426849365234375;0.5465390990314862307286603027023375034332275390625]
      mask Display: e = 0.06;c1 = [120 150 230]/255;c2 = ([120 150 230]+0)/383;c3 = ([120 150 230]+128)/383;patch([0 1 1 0],[0 0 1 1],c1);patch([0 1 1 1-e 1-e 0+e],[0 0 1 1-e 0+e 0+e],c2);patch([0 0 1 1-e 0+e 0+e],[0 1 1 1-e 1-e 0+e],c3);plot([0 1 1 0 0],[0 0 1 1 0]);disp('Weights');
  "IW{1,1}(8,:)'" : Constant  Value=[0.50456389189707928633055189493461512029170989990234375;-0.765140951858942042207445410895161330699920654296875;0.1570690731750348512196779893201892264187335968017578125;0.2681208325762696187410938364337198436260223388671875;-0.82779326613658554823160784508218057453632354736328125;0.356993742779236511442064738730550743639469146728515625;-0.976280129291541509672924803453497588634490966796875;0.16504117848556243419722022736095823347568511962890625;0.356943967948731566419695582226268015801906585693359375;0.66842971143415164103629422243102453649044036865234375;0.449339961286215394675735979035380296409130096435546875;0.14220062142668743465634406675235368311405181884765625]
      mask Display: e = 0.06;c1 = [120 150 230]/255;c2 = ([120 150 230]+0)/383;c3 = ([120 150 230]+128)/383;patch([0 1 1 0],[0 0 1 1],c1);patch([0 1 1 1-e 1-e 0+e],[0 0 1 1-e 0+e 0+e],c2);patch([0 0 1 1-e 0+e 0+e],[0 1 1 1-e 1-e 0+e],c3);plot([0 1 1 0 0],[0 0 1 1 0]);disp('Weights');
  "IW{1,1}(9,:)'" : Constant  Value=[0.7592261612055779540497724156011827290058135986328125;0.046598748903399343779252461672513163648545742034912109375;-0.600588424610740911901984873111359775066375732421875;-0.94958054894314758431761447354801930487155914306640625;-1.3227754501645507811957713784067891538143157958984375;-0.77956703475742183950814023774000816047191619873046875;-0.50440860122289254974248251528479158878326416015625;-0.143701090065957270969221326595288701355457305908203125;0.726324471940543059389483460108749568462371826171875;0.648351302048403521638419988448731601238250732421875;0.6303467404820641828422367325401864945888519287109375;1.24140275687570156293304535211063921451568603515625]
      mask Display: e = 0.06;c1 = [120 150 230]/255;c2 = ([120 150 230]+0)/383;c3 = ([120 150 230]+128)/383;patch([0 1 1 0],[0 0 1 1],c1);patch([0 1 1 1-e 1-e 0+e],[0 0 1 1-e 0+e 0+e],c2);patch([0 0 1 1-e 0+e 0+e],[0 1 1 1-e 1-e 0+e],c3);plot([0 1 1 0 0],[0 0 1 1 0]);disp('Weights');
  Mux : Mux  Inputs=40
      mask Display: e = 0.06;c1 = [120 150 230]/255;c2 = ([120 150 230]+0)/383;c3 = ([120 150 230]+128)/383;patch([0 1 1 0],[0 0 1 1],c1);patch([0 1 1 1-e 1-e 0+e],[0 0 1 1-e 0+e 0+e],c2);patch([0 0 1 1-e 0+e 0+e],[0 1 1 1-e 1-e 0+e],c3);plot([0 1 1 0 0],[0 0 1 1 0]);disp('Mux');
  dotprod{1..40} (40 alike) : neural/Weight Functions/dotprod
  "iz{1,1}" : Outport
      mask Display: e = 0.06;c1 = [120 230 180]/255;c2 = ([120 230 180]+0)/(256+128);c3 = ([120 230 180]+128)/(256+128);patch([0 1 1 0],[0 0 1 1],c1);patch([0 1 1 1-e 1-e 0+e],[0 0 1 1-e 0+e 0+e],c2);patch([0 0 1 1-e 0+e 0+e],[0 1 1 1-e 1-e 0+e],c3);plot([0 1 1 0 0],[0 0 1 1 0]);
  wires:
  "IW{1,1}(1,:)'"/1 -> dotprod1/1
  "pd{1,1}"/1 -> dotprod1/2, dotprod2/2, dotprod3/2, dotprod4/2, dotprod5/2, dotprod6/2, dotprod7/2, dotprod8/2, dotprod9/2, dotprod10/2, dotprod11/2, dotprod12/2, dotprod13/2, dotprod14/2, dotprod15/2, dotprod16/2, dotprod17/2, dotprod18/2, dotprod19/2, dotprod20/2, dotprod21/2, dotprod22/2, dotprod23/2, dotprod24/2, dotprod25/2, dotprod26/2, dotprod27/2, dotprod28/2, dotprod29/2, dotprod30/2, dotprod31/2, dotprod32/2, dotprod33/2, dotprod34/2, dotprod35/2, dotprod36/2, dotprod37/2, dotprod38/2, dotprod39/2, dotprod40/2
  dotprod1/1 -> Mux/1
  "IW{1,1}(2,:)'"/1 -> dotprod2/1
  dotprod2/1 -> Mux/2
  "IW{1,1}(3,:)'"/1 -> dotprod3/1
  dotprod3/1 -> Mux/3
  "IW{1,1}(4,:)'"/1 -> dotprod4/1
  dotprod4/1 -> Mux/4
  "IW{1,1}(5,:)'"/1 -> dotprod5/1
  dotprod5/1 -> Mux/5
  "IW{1,1}(6,:)'"/1 -> dotprod6/1
  dotprod6/1 -> Mux/6
  "IW{1,1}(7,:)'"/1 -> dotprod7/1
  dotprod7/1 -> Mux/7
  "IW{1,1}(8,:)'"/1 -> dotprod8/1
  dotprod8/1 -> Mux/8
  "IW{1,1}(9,:)'"/1 -> dotprod9/1
  dotprod9/1 -> Mux/9
  "IW{1,1}(10,:)'"/1 -> dotprod10/1
  dotprod10/1 -> Mux/10
  "IW{1,1}(11,:)'"/1 -> dotprod11/1
  dotprod11/1 -> Mux/11
  "IW{1,1}(12,:)'"/1 -> dotprod12/1
  dotprod12/1 -> Mux/12
  "IW{1,1}(13,:)'"/1 -> dotprod13/1
  dotprod13/1 -> Mux/13
  "IW{1,1}(14,:)'"/1 -> dotprod14/1
  dotprod14/1 -> Mux/14
  "IW{1,1}(15,:)'"/1 -> dotprod15/1
  dotprod15/1 -> Mux/15
  "IW{1,1}(16,:)'"/1 -> dotprod16/1
  dotprod16/1 -> Mux/16
  "IW{1,1}(17,:)'"/1 -> dotprod17/1
  dotprod17/1 -> Mux/17
  "IW{1,1}(18,:)'"/1 -> dotprod18/1
  dotprod18/1 -> Mux/18
  "IW{1,1}(19,:)'"/1 -> dotprod19/1
  dotprod19/1 -> Mux/19
  "IW{1,1}(20,:)'"/1 -> dotprod20/1
  dotprod20/1 -> Mux/20
  "IW{1,1}(21,:)'"/1 -> dotprod21/1
  dotprod21/1 -> Mux/21
  "IW{1,1}(22,:)'"/1 -> dotprod22/1
  dotprod22/1 -> Mux/22
  "IW{1,1}(23,:)'"/1 -> dotprod23/1
  dotprod23/1 -> Mux/23
  "IW{1,1}(24,:)'"/1 -> dotprod24/1
  dotprod24/1 -> Mux/24
  "IW{1,1}(25,:)'"/1 -> dotprod25/1
  dotprod25/1 -> Mux/25
  "IW{1,1}(26,:)'"/1 -> dotprod26/1
  dotprod26/1 -> Mux/26
  "IW{1,1}(27,:)'"/1 -> dotprod27/1
  dotprod27/1 -> Mux/27
  "IW{1,1}(28,:)'"/1 -> dotprod28/1
  dotprod28/1 -> Mux/28
  "IW{1,1}(29,:)'"/1 -> dotprod29/1
  dotprod29/1 -> Mux/29
  "IW{1,1}(30,:)'"/1 -> dotprod30/1
  dotprod30/1 -> Mux/30
  "IW{1,1}(31,:)'"/1 -> dotprod31/1
  dotprod31/1 -> Mux/31
  "IW{1,1}(32,:)'"/1 -> dotprod32/1
  dotprod32/1 -> Mux/32
  "IW{1,1}(33,:)'"/1 -> dotprod33/1
  dotprod33/1 -> Mux/33
  "IW{1,1}(34,:)'"/1 -> dotprod34/1
  dotprod34/1 -> Mux/34
  "IW{1,1}(35,:)'"/1 -> dotprod35/1
  dotprod35/1 -> Mux/35
  "IW{1,1}(36,:)'"/1 -> dotprod36/1
  dotprod36/1 -> Mux/36
  "IW{1,1}(37,:)'"/1 -> dotprod37/1
  dotprod37/1 -> Mux/37
  "IW{1,1}(38,:)'"/1 -> dotprod38/1
  dotprod38/1 -> Mux/38
  "IW{1,1}(39,:)'"/1 -> dotprod39/1
  dotprod39/1 -> Mux/39
  "IW{1,1}(40,:)'"/1 -> dotprod40/1
  dotprod40/1 -> Mux/40
  Mux/1 -> "iz{1,1}"/1

== system PFE_2Lignes_RNA (2)/RNA_Classificateur/Layer 2/Delays 1 ==
  "p{2}" : Inport  PortDimensions=40
      mask Display: e = 0.06;c1 = [120 230 180]/255;c2 = ([120 230 180]+0)/(256+128);c3 = ([120 230 180]+128)/(256+128);patch([0 1 1 0],[0 0 1 1],c1);patch([0 1 1 1-e 1-e 0+e],[0 0 1 1-e 0+e 0+e],c2);patch([0 0 1 1-e 0+e 0+e],[0 1 1 1-e 1-e 0+e],c3);plot([0 1 1 0 0],[0 0 1 1 0]);
  mux : Mux  Inputs=1
      mask Display: e = 0.06;c1 = [120 150 230]/255;c2 = ([120 150 230]+0)/383;c3 = ([120 150 230]+128)/383;patch([0 1 1 0],[0 0 1 1],c1);patch([0 1 1 1-e 1-e 0+e],[0 0 1 1-e 0+e 0+e],c2);patch([0 0 1 1-e 0+e 0+e],[0 1 1 1-e 1-e 0+e],c3);plot([0 1 1 0 0],[0 0 1 1 0]);disp('Mux')
  "pd{2,1}" : Outport
      mask Display: e = 0.06;c1 = [120 230 180]/255;c2 = ([120 230 180]+0)/(256+128);c3 = ([120 230 180]+128)/(256+128);patch([0 1 1 0],[0 0 1 1],c1);patch([0 1 1 1-e 1-e 0+e],[0 0 1 1-e 0+e 0+e],c2);patch([0 0 1 1-e 0+e 0+e],[0 1 1 1-e 1-e 0+e],c3);plot([0 1 1 0 0],[0 0 1 1 0]);
  wires:
  "p{2}"/1 -> mux/1
  mux/1 -> "pd{2,1}"/1
